simulink model "quadrotor_adrc_simulation_q"  (R2015a)
settings: Solver=ode45  StartTime=0.0  StopTime=10  FixedStep=1e-4  RelTol=1e-4
settings Model: Creator=kbmaj  LastModifiedBy=kbmaj

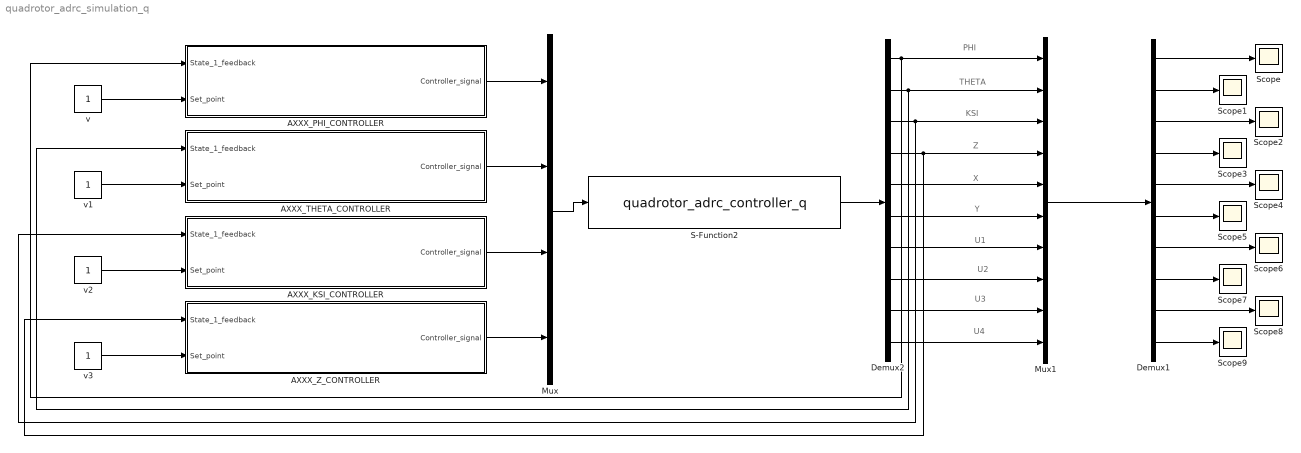
== system quadrotor_adrc_simulation_q ==
  note: U4
  note: U3
  note: U2
  note: U1
  note: Y
  note: X
  note: Z
  note: KSI
  note: THETA
  note: PHI
  AXXX_KSI_CONTROLLER : Subsystem
  AXXX_PHI_CONTROLLER : Subsystem
  AXXX_THETA_CONTROLLER : Subsystem
  AXXX_Z_CONTROLLER : Subsystem
  Demux1 : Demux  Outputs=10
  Demux2 : Demux  Outputs=10
  Mux : Mux
  Mux1 : Mux  Inputs=10
  S-Function2 : S-Function  FunctionName=quadrotor_adrc_controller_q
  Scope{,1..9} (10 alike) : Scope
      Scope2 settings: SaveName=ScopeData2
      Scope3 settings: SaveName=ScopeData3
      Scope4 settings: SaveName=ScopeData4
      Scope5 settings: SaveName=ScopeData5
      Scope6 settings: SaveName=ScopeData6
      Scope7 settings: SaveName=ScopeData7
      Scope8 settings: SaveName=ScopeData8
      Scope9 settings: SaveName=ScopeData9
  v{,1..3} (4 alike) : Constant
  wires:
  S-Function2/1 -> Demux2/1
  Mux/1 -> S-Function2/1
  v/1 -> AXXX_PHI_CONTROLLER/2(Set_point)
  AXXX_PHI_CONTROLLER/1(Controller_signal) -> Mux/1
  v1/1 -> AXXX_THETA_CONTROLLER/2(Set_point)
  AXXX_THETA_CONTROLLER/1(Controller_signal) -> Mux/2
  v2/1 -> AXXX_KSI_CONTROLLER/2(Set_point)
  AXXX_KSI_CONTROLLER/1(Controller_signal) -> Mux/3
  v3/1 -> AXXX_Z_CONTROLLER/2(Set_point)
  AXXX_Z_CONTROLLER/1(Controller_signal) -> Mux/4
  Demux2/10 -> Mux1/10
  Demux2/9 -> Mux1/9
  Demux2/8 -> Mux1/8
  Demux2/7 -> Mux1/7
  Demux2/6 -> Mux1/6
  Demux2/5 -> Mux1/5
  Demux2/4 -> AXXX_Z_CONTROLLER/1(State_1_feedback), Mux1/4
  Demux2/3 -> AXXX_KSI_CONTROLLER/1(State_1_feedback), Mux1/3
  Demux2/2 -> AXXX_THETA_CONTROLLER/1(State_1_feedback), Mux1/2
  Demux2/1 -> AXXX_PHI_CONTROLLER/1(State_1_feedback), Mux1/1
  Mux1/1 -> Demux1/1
  Demux1/1 -> Scope/1
  Demux1/2 -> Scope1/1
  Demux1/3 -> Scope2/1
  Demux1/4 -> Scope3/1
  Demux1/5 -> Scope4/1
  Demux1/6 -> Scope5/1
  Demux1/7 -> Scope6/1
  Demux1/8 -> Scope7/1
  Demux1/9 -> Scope8/1
  Demux1/10 -> Scope9/1

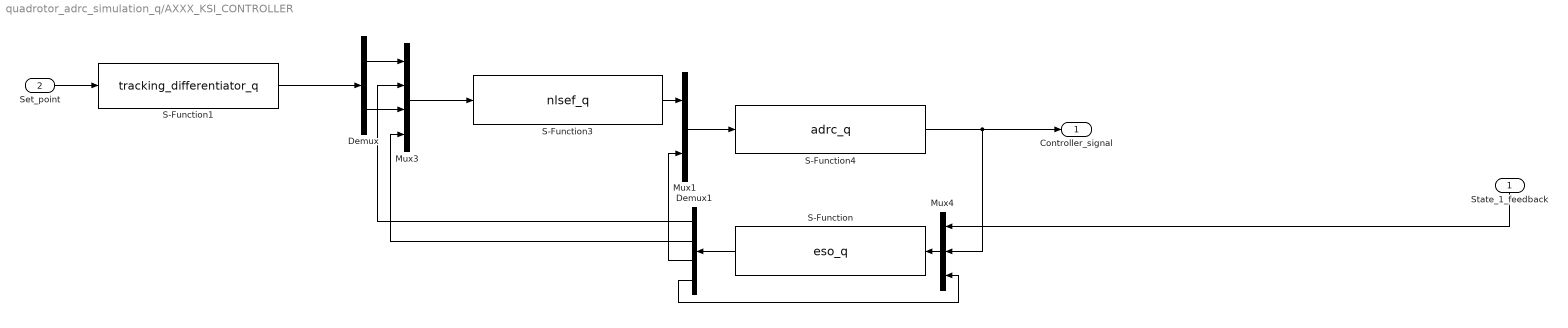
== system quadrotor_adrc_simulation_q/AXXX_KSI_CONTROLLER ==
  State_1_feedback : Inport
  Set_point : Inport  Port=2
  Demux : Demux  Outputs=2
  Demux1 : Demux
  Mux1 : Mux  Inputs=2
  Mux3 : Mux
  Mux4 : Mux  Inputs=3
  S-Function : S-Function  FunctionName=eso_q
  S-Function1 : S-Function  FunctionName=tracking_differentiator_q
  S-Function3 : S-Function  FunctionName=nlsef_q
  S-Function4 : S-Function  FunctionName=adrc_q
  Controller_signal : Outport
  wires:
  S-Function3/1 -> Mux1/1
  Demux1/2 -> Mux3/4
  Demux1/1 -> Mux3/2
  Demux/1 -> Mux3/1
  S-Function4/1 -> Mux4/2, Controller_signal/1
  Demux/2 -> Mux3/3
  Demux1/4 -> Mux4/3
  Set_point/1 -> S-Function1/1
  Mux3/1 -> S-Function3/1
  Mux4/1 -> S-Function/1
  Mux1/1 -> S-Function4/1
  Demux1/3 -> Mux1/2
  S-Function/1 -> Demux1/1
  S-Function1/1 -> Demux/1
  State_1_feedback/1 -> Mux4/1

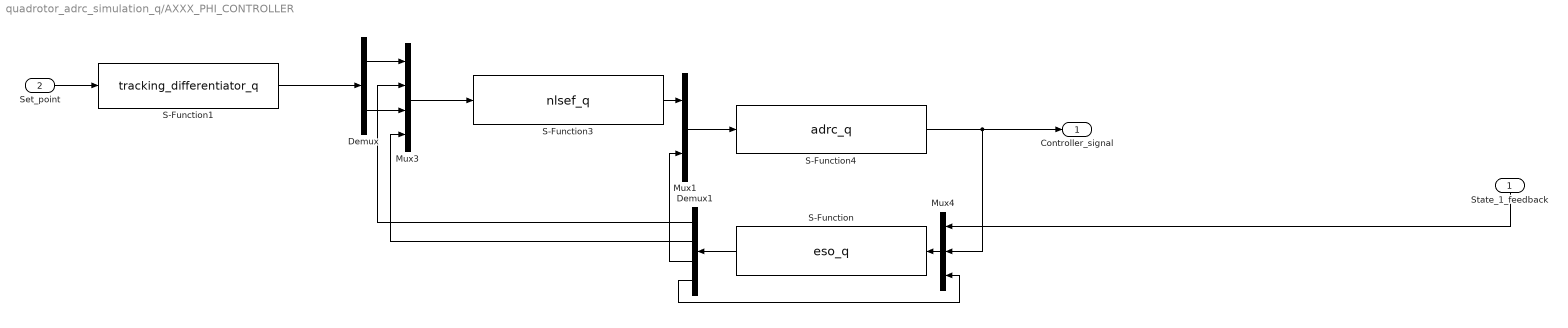
== system quadrotor_adrc_simulation_q/AXXX_PHI_CONTROLLER ==
  State_1_feedback : Inport
  Set_point : Inport  Port=2
  Demux : Demux  Outputs=2
  Demux1 : Demux
  Mux1 : Mux  Inputs=2
  Mux3 : Mux
  Mux4 : Mux  Inputs=3
  S-Function : S-Function  FunctionName=eso_q
  S-Function1 : S-Function  FunctionName=tracking_differentiator_q
  S-Function3 : S-Function  FunctionName=nlsef_q
  S-Function4 : S-Function  FunctionName=adrc_q
  Controller_signal : Outport
  wires:
  S-Function3/1 -> Mux1/1
  Demux1/2 -> Mux3/4
  Demux1/1 -> Mux3/2
  Demux/1 -> Mux3/1
  S-Function4/1 -> Mux4/2, Controller_signal/1
  Demux/2 -> Mux3/3
  Demux1/4 -> Mux4/3
  Set_point/1 -> S-Function1/1
  Mux3/1 -> S-Function3/1
  Mux4/1 -> S-Function/1
  Mux1/1 -> S-Function4/1
  Demux1/3 -> Mux1/2
  S-Function/1 -> Demux1/1
  S-Function1/1 -> Demux/1
  State_1_feedback/1 -> Mux4/1

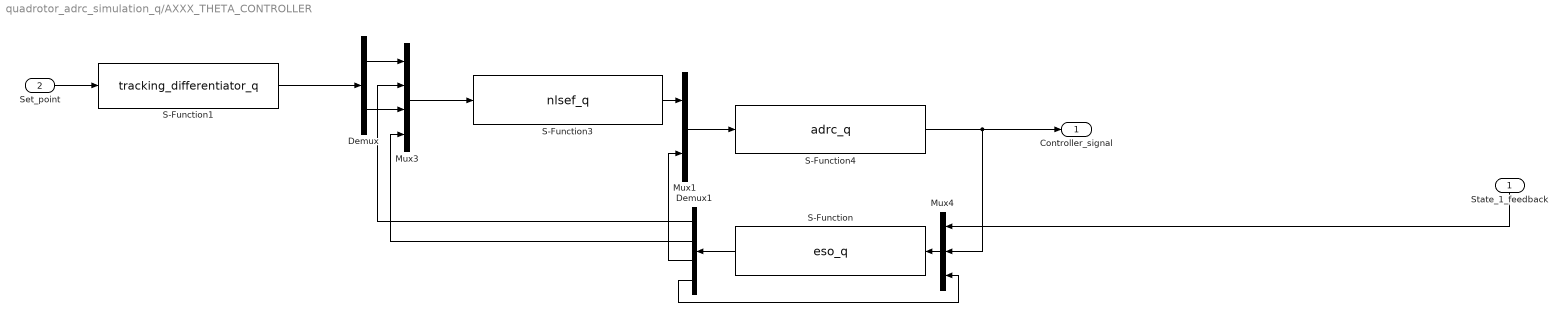
== system quadrotor_adrc_simulation_q/AXXX_THETA_CONTROLLER ==
  State_1_feedback : Inport
  Set_point : Inport  Port=2
  Demux : Demux  Outputs=2
  Demux1 : Demux
  Mux1 : Mux  Inputs=2
  Mux3 : Mux
  Mux4 : Mux  Inputs=3
  S-Function : S-Function  FunctionName=eso_q
  S-Function1 : S-Function  FunctionName=tracking_differentiator_q
  S-Function3 : S-Function  FunctionName=nlsef_q
  S-Function4 : S-Function  FunctionName=adrc_q
  Controller_signal : Outport
  wires:
  S-Function3/1 -> Mux1/1
  Demux1/2 -> Mux3/4
  Demux1/1 -> Mux3/2
  Demux/1 -> Mux3/1
  S-Function4/1 -> Mux4/2, Controller_signal/1
  Demux/2 -> Mux3/3
  Demux1/4 -> Mux4/3
  Set_point/1 -> S-Function1/1
  Mux3/1 -> S-Function3/1
  Mux4/1 -> S-Function/1
  Mux1/1 -> S-Function4/1
  Demux1/3 -> Mux1/2
  S-Function/1 -> Demux1/1
  S-Function1/1 -> Demux/1
  State_1_feedback/1 -> Mux4/1

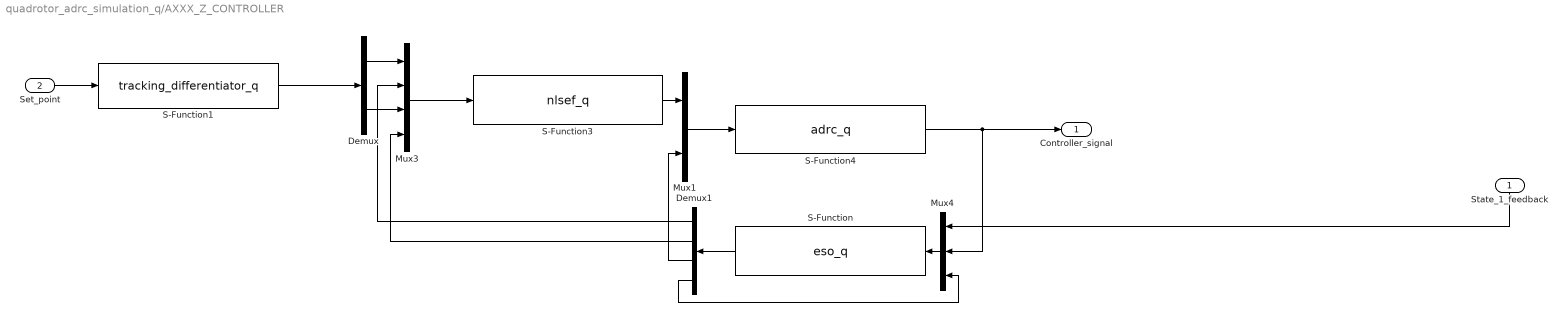
== system quadrotor_adrc_simulation_q/AXXX_Z_CONTROLLER ==
  State_1_feedback : Inport
  Set_point : Inport  Port=2
  Demux : Demux  Outputs=2
  Demux1 : Demux
  Mux1 : Mux  Inputs=2
  Mux3 : Mux
  Mux4 : Mux  Inputs=3
  S-Function : S-Function  FunctionName=eso_q
  S-Function1 : S-Function  FunctionName=tracking_differentiator_q
  S-Function3 : S-Function  FunctionName=nlsef_q
  S-Function4 : S-Function  FunctionName=adrc_q
  Controller_signal : Outport
  wires:
  S-Function3/1 -> Mux1/1
  Demux1/2 -> Mux3/4
  Demux1/1 -> Mux3/2
  Demux/1 -> Mux3/1
  S-Function4/1 -> Mux4/2, Controller_signal/1
  Demux/2 -> Mux3/3
  Demux1/4 -> Mux4/3
  Set_point/1 -> S-Function1/1
  Mux3/1 -> S-Function3/1
  Mux4/1 -> S-Function/1
  Mux1/1 -> S-Function4/1
  Demux1/3 -> Mux1/2
  S-Function/1 -> Demux1/1
  S-Function1/1 -> Demux/1
  State_1_feedback/1 -> Mux4/1
